simulink model "gain_scheduled_control_simulink_model"  (R2022b)
settings: Solver=VariableStepAuto  StartTime=0.0  StopTime=900  RelTol=1e-3
values from neighbouring files (symbols this model uses):
  A_tem = 0.001^2    (= 1e-06)    [model_parameters.m]
  Cap_sink_bottom = m_sink_bottom*c_sink_bottom    (= 585)    [model_parameters.m]
  Cap_sink_top = m_sink_top*c_sink_top    (= 153)    [model_parameters.m]
  Km = 8.48e-3    (= 0.00848)    [model_parameters.m]
  L = 2e-3    (= 0.002)    [model_parameters.m]
  R_sink_bottom = 0.16    [model_parameters.m]
  R_sink_top = 0.5    [model_parameters.m]
  R_wall = (w/(k_wall*A_wall))    (= 7.79727095517)    [model_parameters.m]
  Rm = 3.05    [model_parameters.m]
  Sm = 0.546    [model_parameters.m]
  T_amb = 23    [model_parameters.m]
  temp = [18]    [model_linearization.m]
undefined symbols (not defined in the file or in its folder): controllers
libraries: slpidlib x1
settings Model: Creator=User  LastModifiedBy=User

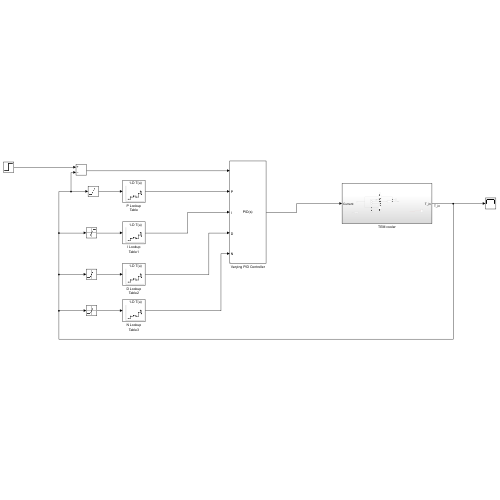
[thumbnail: Simulink's stored preview of the top-level diagram]
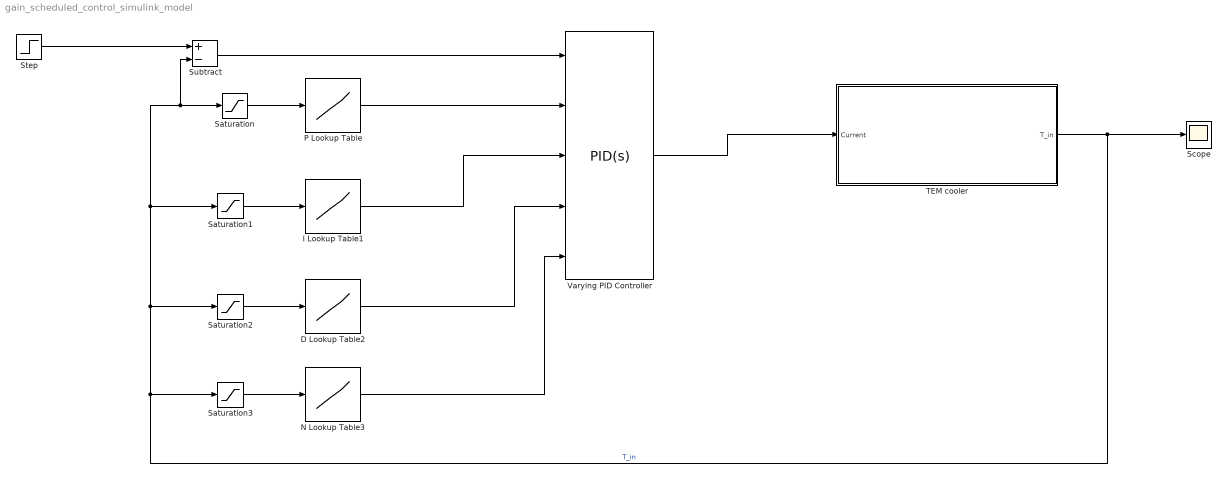
== system gain_scheduled_control_simulink_model ==
  D Lookup Table2 : Lookup_n-D  NumberOfTableDimensions=1  LookupTableObject=''  BreakpointsForDimension1=temp  BreakpointsForDimension2=[1:2]  BreakpointsForDimension3=[5, 7]  BreakpointsForDimension1FirstPoint=10  BreakpointsForDimension2FirstPoint=10  BreakpointsForDimension1Spacing=12  BreakpointsForDimension2Spacing=12  IndexSearchMethod=Evenly spaced points  Table=controllers.KD  InterpMethod=Flat  DiagnosticForOutOfRangeInput=Error  InternalRulePriority=Speed  RndMeth=Simplest
  I Lookup Table1 : Lookup_n-D  NumberOfTableDimensions=1  LookupTableObject=''  BreakpointsForDimension1=temp  BreakpointsForDimension2=[1:2]  BreakpointsForDimension3=[5, 7]  BreakpointsForDimension1FirstPoint=10  BreakpointsForDimension2FirstPoint=10  BreakpointsForDimension1Spacing=12  BreakpointsForDimension2Spacing=12  IndexSearchMethod=Evenly spaced points  Table=controllers.KI  InterpMethod=Flat  DiagnosticForOutOfRangeInput=Error  InternalRulePriority=Speed  RndMeth=Simplest
  N Lookup Table3 : Lookup_n-D  NumberOfTableDimensions=1  LookupTableObject=''  BreakpointsForDimension1=temp  BreakpointsForDimension2=[1:2]  BreakpointsForDimension3=[5, 7]  BreakpointsForDimension1FirstPoint=10  BreakpointsForDimension2FirstPoint=10  BreakpointsForDimension1Spacing=12  BreakpointsForDimension2Spacing=12  IndexSearchMethod=Evenly spaced points  Table=controllers.Tf  InterpMethod=Flat  DiagnosticForOutOfRangeInput=Error  InternalRulePriority=Speed  RndMeth=Simplest
  P Lookup Table : Lookup_n-D  NumberOfTableDimensions=1  LookupTableObject=''  BreakpointsForDimension1=temp  BreakpointsForDimension2=[1:2]  BreakpointsForDimension3=[5, 7]  BreakpointsForDimension1FirstPoint=10  BreakpointsForDimension2FirstPoint=10  BreakpointsForDimension1Spacing=12  BreakpointsForDimension2Spacing=12  IndexSearchMethod=Evenly spaced points  Table=controllers.Kp  InterpMethod=Flat  DiagnosticForOutOfRangeInput=Error  InternalRulePriority=Speed  RndMeth=Simplest
  Saturation{,1..3} (4 alike) : Saturate  UpperLimit=23  LowerLimit=8
  Scope : Scope
  Step : Step  Time=0  After=18  SampleTime=0
  Subtract : Sum  Inputs=+-
  TEM cooler : Subsystem
  Varying PID Controller : slpidlib/PID Controller  Controller=PID  Form=Parallel  TimeDomain=Continuous-time  UseExternalTs=off  SampleTime=-1  IntegratorMethod=Forward Euler  FilterMethod=Forward Euler  ControllerParametersSource=external  P=1  I=1  UseKiTs=off  D=0  N=100  UseFilter=on  TunerSelectOption=Transfer Function Based (PID Tuner App)  InitialConditionSource=internal  InitialConditionForIntegrator=0  InitialConditionForFilter=0  DifferentiatorICPrevScaledInput=0  ExternalReset=none  TrackingMode=off  Kt=1  LimitOutput=off  SatLimitsSource=internal  UpperSaturationLimit=inf  LowerSaturationLimit=-inf  LinearizeAsGain=on  AntiWindupMode=none  Kb=1  LimitIntegrator=off  UpperIntegratorSaturationLimit=inf  LowerIntegratorSaturationLimit=-inf  POutMin=[]  POutMax=[]  IOutMin=[]  IOutMax=[]  DOutMin=[]  DOutMax=[]  NOutMin=[]  NOutMax=[]  SumOutMin=[]  SumOutMax=[]  SaturationOutMin=[]  SaturationOutMax=[]  PParamMin=[]  PParamMax=[]  IParamMin=[]  IParamMax=[]  DParamMin=[]  DParamMax=[]  NParamMin=[]  NParamMax=[]  KbParamMin=[]  KbParamMax=[]  KtParamMin=[]  KtParamMax=[]  KbOutMin=[]  KbOutMax=[]  KtOutMin=[]  KtOutMax=[]  IntegratorOutMin=[]  IntegratorOutMax=[]  FilterOutMin=[]  FilterOutMax=[]  SumI1OutMin=[]  SumI1OutMax=[]  SumI2OutMin=[]  SumI2OutMax=[]  SumI3OutMin=[]  SumI3OutMax=[]  SumI4OutMin=[]  SumI4OutMax=[]  SumDOutMin=[]  SumDOutMax=[]  DifferentiatorOutMin=[]  DifferentiatorOutMax=[]  FilterDiffOutCoefMin=[]  FilterDiffOutCoefMax=[]  ReciprocalOutMin=[]  ReciprocalOutMax=[]  SumDenOutMin=[]  SumDenOutMax=[]  SumNumOutMin=[]  SumNumOutMax=[]  DivideOutMin=[]  DivideOutMax=[]  UdiffTsProdOutMin=[]  UdiffTsProdOutMax=[]  NTsProdOutMin=[]  NTsProdOutMax=[]  UintegralTsProdOutMin=[]  UintegralTsProdOutMax=[]  UngainTsProdOutMin=[]  UngainTsProdOutMax=[]  ClampingZeroOutDataTypeStr=Inherit: Inherit via back propagation  ClampingZeroOutMin=[]  ClampingZeroOutMax=[]  FilterDenConstantOutDataTypeStr=Inherit: Inherit via back propagation  FilterDenConstantOutMin=[]  FilterDenConstantOutMax=[]  PCopyOutDataTypeStr=Inherit: Inherit via back propagation  PCopyOutMin=[]  PCopyOutMax=[]  NCopyOutDataTypeStr=Inherit: Inherit via back propagation  NCopyOutMin=[]  NCopyOutMax=[]  IntegratorContinuousStateAttributes=''  IntegratorStateMustResolveToSignalObject=off  IntegratorRTWStateStorageClass=Auto  FilterContinuousStateAttributes=''  FilterStateMustResolveToSignalObject=off  FilterRTWStateStorageClass=Auto  ParallelPVariant=ExternalParameters  IdealPVariant=Disabled  IVariant=ExternalParameters  DVariant=ExternalParameters  IntegratorVariant=Continuous  SatVariant=Disabled  AWVariant=Passthrough  PCopyVariant=Disabled  TRVariant=Disabled  FdbkBlocksVariant=Forward  IdealPFdbkVariant=Disabled  SatFdbkVariant=Disabled  DerivativeFilterVariant=ContFilter  NVariant=ExternalParameters  NCopyVariant=Disabled  FilterICVariant=InternalICsFilter  IntegratorICVariant=InternalICs  ExternalResetVariant=Disabled  TRSumVariant=Passthrough  SumFdbkVariant=Disabled  SumVariant=Sum_PID  TsampFilterVariant=InternalTs  TsampNgainVariant=Passthrough  TsampIntegralVariant=Passthrough  ExternalSaturationOutDataTypeStr=Inherit: Same as second input
      settings: LibrarySourceBlock=cstblocks/Linear Parameter Varying/Varying PID Controller
  wires:
  Varying PID Controller/1 -> TEM cooler/1(Current)
  TEM cooler/1(T_in) -> Saturation2/1, Subtract/2, Saturation/1, Saturation1/1, Saturation3/1, Scope/1  "T_in"
  I Lookup Table1/1 -> Varying PID Controller/3
  D Lookup Table2/1 -> Varying PID Controller/4
  P Lookup Table/1 -> Varying PID Controller/2
  N Lookup Table3/1 -> Varying PID Controller/5
  Step/1 -> Subtract/1
  Subtract/1 -> Varying PID Controller/1
  Saturation/1 -> P Lookup Table/1
  Saturation1/1 -> I Lookup Table1/1
  Saturation2/1 -> D Lookup Table2/1
  Saturation3/1 -> N Lookup Table3/1

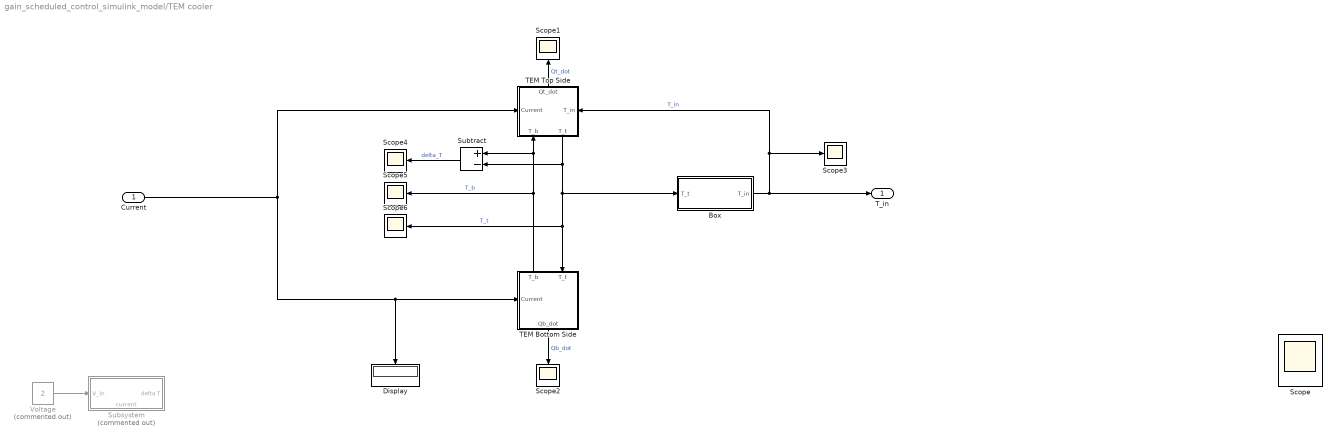
== system gain_scheduled_control_simulink_model/TEM cooler ==
  Current : Inport
  Box : Subsystem
  Display : Display
  Scope{,1..6} (7 alike) : Scope
  Subsystem : Subsystem  Commented=on
      settings: PortSchema="{\"entries\":[{\"content\":{\"sides\":[{\"content\":{\"connectorIds\":[\"In1\"]},\"type\":\"ConnectorPlacement.EquallySpacedRectSide\",\"uuid\":\"bf310b45-256c-480b-87aa-4ce33626a7e5\"},{\"content\":{\"connectorIds\":[\"In2\"],\"side\":\"RIGHT\"},\"type\":\"ConnectorPlacement.EquallySpacedRectSide\",\"uuid\":\"b70f7f05-59db-424a-a94e-53d826ff0d1d\"},{\"content\":{\"connectorIds\":[],\"side\":\"TOP\"},\"type\":\"ConnectorPlacement.EquallySpacedRectSide\",\"uuid\":\"289579d9-4cfd-4dc6-b96e-4dd4bd82e132\"},{\"content\":{\"connectorIds\":[\"Out1\"],\"side\":\"BOTTOM\"},\"type\":\"ConnectorPlacement.EquallySpacedRectSide\",\"uuid\":\"73a9f64e-8cf6-43a0-a8cf-b599e511ce8d\"}]},\"type\":\"ConnectorPlacement.EquallySpacedConnector\",\"uuid\":\"06e6aee1-3e48-43b7-820b-fcdb22568c21\"}],\"packageUris\":[\"http://schema.mathworks.com/mf0/Connector/R2020b\"],\"version\":\"1.0\"}"
  Subtract : Sum  Inputs=+-
  TEM Bottom Side : Subsystem
      settings: PortSchema="{\"entries\":[{\"content\":{\"sides\":[{\"content\":{\"connectorIds\":[\"In1\"]},\"type\":\"ConnectorPlacement.EquallySpacedRectSide\",\"uuid\":\"b87a4581-d8f8-4fc9-b563-d914d24460f9\"},{\"content\":{\"connectorIds\":[],\"side\":\"RIGHT\"},\"type\":\"ConnectorPlacement.EquallySpacedRectSide\",\"uuid\":\"1ae113cc-1538-4d91-9da7-a2b119848b58\"},{\"content\":{\"connectorIds\":[\"Out2\",\"In2\"],\"side\":\"TOP\"},\"type\":\"ConnectorPlacement.EquallySpacedRectSide\",\"uuid\":\"f7878c0a-e050-464b-882f-e0962183bf20\"},{\"content\":{\"connectorIds\":[\"Out1\"],\"side\":\"BOTTOM\"},\"type\":\"ConnectorPlacement.EquallySpacedRectSide\",\"uuid\":\"7cf61646-da49-46e9-ae5b-a07c7e6c0ea7\"}]},\"type\":\"ConnectorPlacement.EquallySpacedConnector\",\"uuid\":\"98b85d6f-8037-419b-8688-659007a86e84\"}],\"packageUris\":[\"http://schema.mathworks.com/mf0/Connector/R2020b\"],\"version\":\"1.0\"}"
  TEM Top Side : Subsystem
      settings: PortSchema="{\"entries\":[{\"content\":{\"sides\":[{\"content\":{\"connectorIds\":[\"In1\"]},\"type\":\"ConnectorPlacement.EquallySpacedRectSide\",\"uuid\":\"b87a4581-d8f8-4fc9-b563-d914d24460f9\"},{\"content\":{\"connectorIds\":[\"In3\"],\"side\":\"RIGHT\"},\"type\":\"ConnectorPlacement.EquallySpacedRectSide\",\"uuid\":\"1ae113cc-1538-4d91-9da7-a2b119848b58\"},{\"content\":{\"connectorIds\":[\"Out2\"],\"side\":\"TOP\"},\"type\":\"ConnectorPlacement.EquallySpacedRectSide\",\"uuid\":\"f7878c0a-e050-464b-882f-e0962183bf20\"},{\"content\":{\"connectorIds\":[\"In2\",\"Out1\"],\"side\":\"BOTTOM\"},\"type\":\"ConnectorPlacement.EquallySpacedRectSide\",\"uuid\":\"483b5ab4-c148-4c7c-8dd9-8b046b2eea20\"}]},\"type\":\"ConnectorPlacement.EquallySpacedConnector\",\"uuid\":\"98b85d6f-8037-419b-8688-659007a86e84\"}],\"packageUris\":[\"http://schema.mathworks.com/mf0/Connector/R2020b\"],\"version\":\"1.0\"}"
  Voltage : Constant  Commented=on  Value=2
  T_in : Outport
  wires:
  ? -> Scope/1
  TEM Top Side/1(T_t) -> Box/1(T_t), TEM Bottom Side/2(T_t), Scope6/1, Subtract/2  "T_t"
  TEM Bottom Side/2(T_b) -> Scope5/1, Subtract/1, TEM Top Side/2(T_b)  "T_b"
  TEM Top Side/2(Qt_dot) -> Scope1/1  "Qt_dot"
  TEM Bottom Side/1(Qb_dot) -> Scope2/1  "Qb_dot"
  Box/1(T_in) -> T_in/1, Scope3/1, TEM Top Side/3(T_in)  "T_in"
  Subtract/1 -> Scope4/1  "delta_T"
  Voltage/1 -> Subsystem/1(V_in)
  Current/1 -> TEM Top Side/1(Current), Display/1, TEM Bottom Side/1(Current)

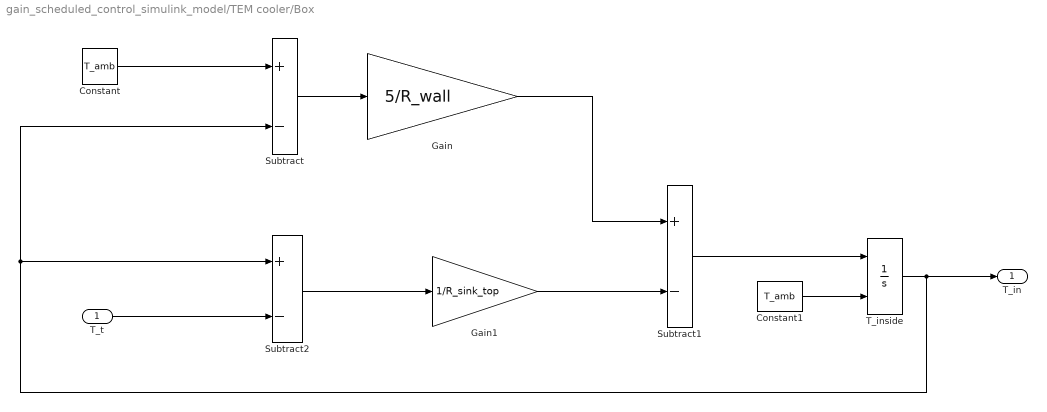
== system gain_scheduled_control_simulink_model/TEM cooler/Box ==
  T_t : Inport
  Constant : Constant  Value=T_amb
  Constant1 : Constant  Value=T_amb
  Gain : Gain  Gain=5/R_wall
  Gain1 : Gain  Gain=1/R_sink_top
  Subtract : Sum  Inputs=+-
  Subtract1 : Sum  Inputs=+-
  Subtract2 : Sum  Inputs=+-
  T_inside : Integrator  InitialConditionSource=external
  T_in : Outport
  wires:
  Constant/1 -> Subtract/1
  T_inside/1 -> T_in/1, Subtract2/1, Subtract/2
  Subtract/1 -> Gain/1
  Gain/1 -> Subtract1/1
  T_t/1 -> Subtract2/2
  Subtract1/1 -> T_inside/1
  Constant1/1 -> T_inside/2
  Subtract2/1 -> Gain1/1
  Gain1/1 -> Subtract1/2

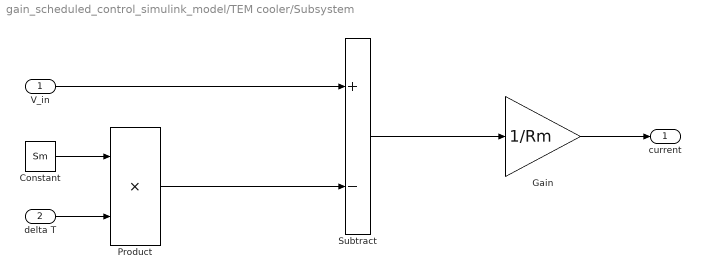
== system gain_scheduled_control_simulink_model/TEM cooler/Subsystem ==
  V_in : Inport
  delta T : Inport  Port=2
  Constant : Constant  Value=Sm
  Gain : Gain  Gain=1/Rm
  Product : Product
  Subtract : Sum  Inputs=+-
  current : Outport
  wires:
  V_in/1 -> Subtract/1
  Constant/1 -> Product/1
  delta T/1 -> Product/2
  Product/1 -> Subtract/2
  Subtract/1 -> Gain/1
  Gain/1 -> current/1

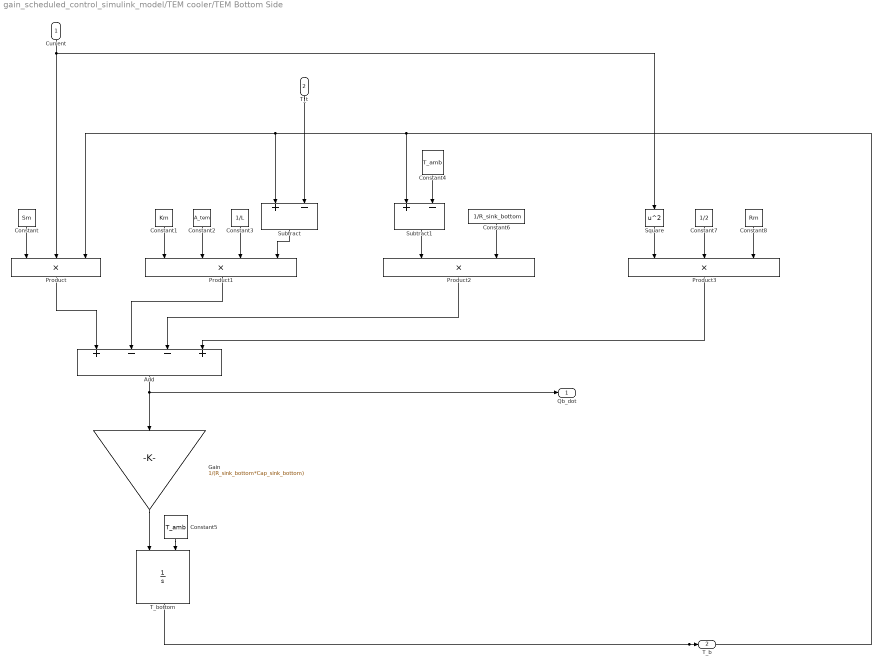
== system gain_scheduled_control_simulink_model/TEM cooler/TEM Bottom Side ==
  Current : Inport
  T_t : Inport  Port=2
  Add : Sum  Inputs=+--+
  Constant : Constant  Value=Sm
  Constant1 : Constant  Value=Km
  Constant2 : Constant  Value=A_tem
  Constant3 : Constant  Value=1/L
  Constant4 : Constant  Value=T_amb
  Constant5 : Constant  Value=T_amb
  Constant6 : Constant  Value=1/R_sink_bottom
  Constant7 : Constant  Value=1/2
  Constant8 : Constant  Value=Rm
  Gain : Gain  Gain=1/(R_sink_bottom*Cap_sink_bottom)
  Product : Product  Inputs=3
  Product1 : Product  Inputs=4
  Product2 : Product
  Product3 : Product  Inputs=3
  Square : Math  Operator=square
  Subtract : Sum  Inputs=+-
  Subtract1 : Sum  Inputs=+-
  T_bottom : Integrator  InitialConditionSource=external
  Qb_dot : Outport
  T_b : Outport  Port=2
  wires:
  Constant/1 -> Product/1
  Constant1/1 -> Product1/1
  Constant2/1 -> Product1/2
  Constant3/1 -> Product1/3
  Subtract/1 -> Product1/4
  Product/1 -> Add/1
  Product1/1 -> Add/2
  Add/1 -> Gain/1, Qb_dot/1
  Gain/1 -> T_bottom/1
  Constant5/1 -> T_bottom/2
  T_bottom/1 -> T_b/1, Product/3, Subtract/1, Subtract1/1
  T_t/1 -> Subtract/2
  Subtract1/1 -> Product2/1
  Constant4/1 -> Subtract1/2
  Constant6/1 -> Product2/2
  Product2/1 -> Add/3
  Current/1 -> Square/1, Product/2
  Constant7/1 -> Product3/2
  Square/1 -> Product3/1
  Constant8/1 -> Product3/3
  Product3/1 -> Add/4

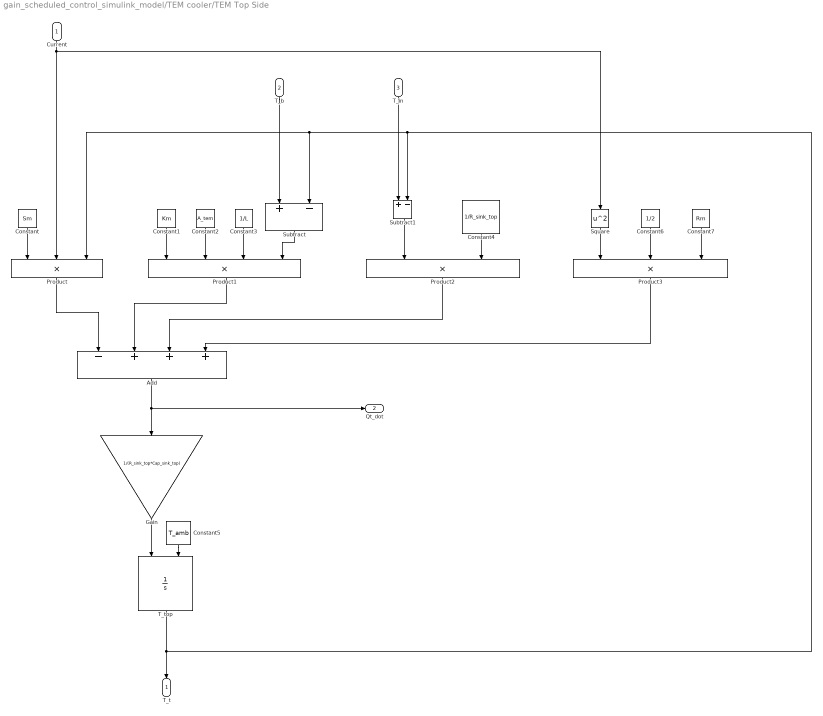
== system gain_scheduled_control_simulink_model/TEM cooler/TEM Top Side ==
  Current : Inport
  T_b : Inport  Port=2
  T_in : Inport  Port=3
  Add : Sum  Inputs=-+++
  Constant : Constant  Value=Sm
  Constant1 : Constant  Value=Km
  Constant2 : Constant  Value=A_tem
  Constant3 : Constant  Value=1/L
  Constant4 : Constant  Value=1/R_sink_top
  Constant5 : Constant  Value=T_amb
  Constant6 : Constant  Value=1/2
  Constant7 : Constant  Value=Rm
  Gain : Gain  Gain=1/(R_sink_top*Cap_sink_top)
  Product : Product  Inputs=3
  Product1 : Product  Inputs=4
  Product2 : Product
  Product3 : Product  Inputs=3
  Square : Math  Operator=square
  Subtract : Sum  Inputs=+-
  Subtract1 : Sum  Inputs=+-
  T_top : Integrator  InitialConditionSource=external
  T_t : Outport
  Qt_dot : Outport  Port=2
  wires:
  Current/1 -> Product/2, Square/1
  Constant/1 -> Product/1
  Constant1/1 -> Product1/1
  Constant2/1 -> Product1/2
  Constant3/1 -> Product1/3
  Subtract/1 -> Product1/4
  Product/1 -> Add/1
  Product1/1 -> Add/2
  Add/1 -> Qt_dot/1, Gain/1
  Gain/1 -> T_top/1
  Constant5/1 -> T_top/2
  T_top/1 -> Subtract1/2, Product/3, Subtract/2, T_t/1
  T_b/1 -> Subtract/1
  Constant4/1 -> Product2/2
  T_in/1 -> Subtract1/1
  Subtract1/1 -> Product2/1
  Product2/1 -> Add/3
  Square/1 -> Product3/1
  Constant6/1 -> Product3/2
  Constant7/1 -> Product3/3
  Product3/1 -> Add/4
